simulink library "bcm"  (R2021b)
settings: Solver=VariableStepAuto  StartTime=0.0  StopTime=10.0  RelTol=1e-3
undefined symbols (not defined in the file or in its folder): KBCM_BSDFlashOFFT_cnt, KBCM_BSDFlashONT_cnt, KBCM_BSDRedMode_enum, KBCM_BSDWarnReqLv_enum, KBCM_FireBuzzerEN_flg, KBCM_FLTurnLPLv_A, KBCM_FRTurnLPLv_A, KBCM_LampOFFV_V, KBCM_LampONV_V, KBCM_LightDelayOFFT_Cnt, KBCM_LightDelayONT_Cnt, KBCM_RLTurnLPLv_A, KBCM_RRTurnLPLv_A
libraries: simulink x103, hdlsllib x1
(part 1 of 3)
settings Model: Creator=user  LastModifiedBy=FVT22063
settings SolverCC: AlgebraicLoopSolver=TrustRegion
settings DebuggingCC: SFMachineParentedDataDiag=warning

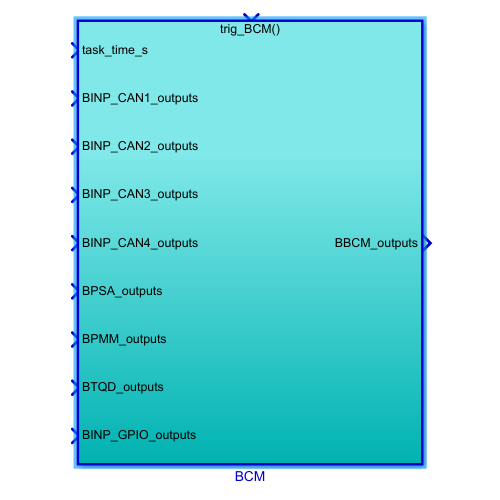
[thumbnail: Simulink's stored preview of the top-level diagram]
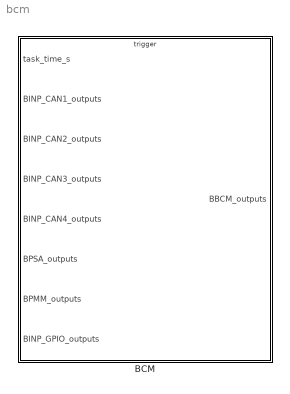
== system bcm ==
  BCM : Subsystem  TreatAsAtomicUnit=on
      settings: RTWSystemCode=Nonreusable function  RTWFcnNameOpts=Use subsystem name  RTWFileNameOpts=Use subsystem name

== system bcm/BCM ==
  note: WarnLv/Mode will be updated on CMM next ver
  note: (Reserved)
      | Actual hazardSW is combinded by L/RTurnSW
  task_time_s : Inport
  BINP_CAN1_outputs : Inport  Port=2  OutDataTypeStr=Bus: BINP_CAN1_outputs
  BINP_CAN2_outputs : Inport  Port=3  OutDataTypeStr=Bus: BINP_CAN2_outputs
  BINP_CAN3_outputs : Inport  Port=4  OutDataTypeStr=Bus: BINP_CAN3_outputs
  BINP_CAN4_outputs : Inport  Port=5  OutDataTypeStr=Bus: BINP_CAN4_outputs
  BPSA_outputs : Inport  Port=6  OutDataTypeStr=Bus: BPSA_outputs
  BPMM_outputs : Inport  Port=7  OutDataTypeStr=Bus: BPMM_outputs
  BINP_GPIO_outputs : Inport  Port=8  OutDataTypeStr=Bus: BINP_GPIO_outputs
  trig_BCM : TriggerPort  TriggerType=function-call  VariantControl=(inherit)
  BBCM_outputs33 : BusCreator  Inputs=56  OutDataTypeStr=Bus: BBCM_outputs  NonVirtualBus=on
  Bus Selector1 : BusSelector  OutputSignals=VINP_EmergencyExitSW_flg,VINP_OSDoorSwOpen_flg,VINP_OSDoorSwClose_flg,VINP_RightTurnSW_flg,VINP_LeftTurnSW_flg
  Bus Selector15 : BusSelector  OutputSignals=VPSA_Keystatus_enum
  Bus Selector16 : BusSelector  OutputSignals=VINP_ZFRBCMHeadLpSWSta_flg,VINP_ZFRBCMHBeamSWSta_flg,VINP_ZFRBCMAutoLightSWSta_flg,VINP_ZFRBCMLightSensorVSta_V,VINP_ZFRBCMPLampSta_flg,VINP_ZFRBCMLFTurnLpCSta_A,VINP_ZFRBCMRFTurnLpCSta_A,VINP_ZRRBCMLRTurnLpCSta_A,VINP_ZRRBCMRRTurnLpCSta_A,VINP_ZRRBCMSTOPSWSta_flg,VINP_ZRRBCMSTOPSW2Sta_flg,VINP_ZRRBCMCallingSWSta_flg,VINP_ZFRBCMWiperASSta_flg,VINP_ZFRBCMWiperHSWSta_flg,VINP_ZFRBCMWiperLSWSta_flg,VINP_ZFRBCMWasherSWSta_flg,VINP_ZFRBCMRFogLpSWSta_flg
  Bus Selector17 : BusSelector  OutputSignals=VPMM_HVILFail_flg
  Bus Selector18 : BusSelector  OutputSignals=VINP_FASpeed_kph,VINP_EBSBrakeSw_enum
  Bus Selector19 : BusSelector  OutputSignals=VINP_B2VFaultCode_enum
  Cast To Boolean : DataTypeConversion  OutDataTypeStr=boolean
  Ground : Ground
  Model Info : simulink/Model-Wide Utilities/Model Info  Frame=on  DisplayStringWithTags=$Id: pmm.mdl 130 2021-02-08 12:40:01Z Shawn $  HorizontalTextAlignment=Center  LeftAlignmentValue=0.5
  Subsystem : Subsystem
  Terminator1 : Terminator
  BBCM_outputs : Outport  OutDataTypeStr=Bus: BBCM_outputs  VectorParamsAs1DForOutWhenUnconnected=off
  wires:
  BPSA_outputs/1 -> Bus Selector15/1
  Bus Selector15/1 -> Subsystem/1(VPMM_VCUKeyStatus_enum)  "<VPSA_Keystatus_enum>"
  BINP_CAN4_outputs/1 -> Bus Selector16/1
  Bus Selector16/1 -> Subsystem/3(VINP_ZFRBCMHeadLpSWSta_flg)  "<VINP_ZFRBCMHeadLpSWSta_flg>"
  Bus Selector16/2 -> Subsystem/4(VINP_ZFRBCMHBeamSWSta_flg)  "<VINP_ZFRBCMHBeamSWSta_flg>"
  Bus Selector16/3 -> Subsystem/5(VINP_ZFRBCMAutoLightSWSta_flg)  "<VINP_ZFRBCMAutoLightSWSta_flg>"
  Bus Selector16/4 -> Subsystem/6(VINP_ZFRBCMLightSensorVSta_V)  "<VINP_ZFRBCMLightSensorVSta_V>"
  Bus Selector16/5 -> Subsystem/7(VINP_ZFRBCMPosLpSWSta_flg)  "<VINP_ZFRBCMPLampSta_flg>"
  Bus Selector16/6 -> Subsystem/8(VINP_ZFRBCMLFTurnLpCSta_A)  "<VINP_ZFRBCMLFTurnLpCSta_A>"
  Bus Selector16/7 -> Subsystem/9(VINP_ZFRBCMRFTurnLpCSta_A)  "<VINP_ZFRBCMRFTurnLpCSta_A>"
  Bus Selector16/8 -> Subsystem/10(VINP_ZRRBCMLRTurnLpCSta_A)  "<VINP_ZRRBCMLRTurnLpCSta_A>"
  Bus Selector16/9 -> Subsystem/11(VINP_ZRRBCMRRTurnLpCSta_A)  "<VINP_ZRRBCMRRTurnLpCSta_A>"
  Ground/1 -> Cast To Boolean/1
  Cast To Boolean/1 -> Subsystem/59(VINP_HazardSW_flg)
  BPMM_outputs/1 -> Bus Selector17/1
  Bus Selector17/1 -> Subsystem/2(VINP_VCUHVILSta_flg)  "<VPMM_HVILFail_flg>"
  Bus Selector16/10 -> Subsystem/12(VINP_ZRRBCMSTOPSWSta_flg)  "<VINP_ZRRBCMSTOPSWSta_flg>"
  Bus Selector16/11 -> Subsystem/13(VINP_ZRRBCMSTOPSW2Sta_flg)  "<VINP_ZRRBCMSTOPSW2Sta_flg>"
  Bus Selector16/12 -> Subsystem/14(VINP_ZRRBCMCallingSWSta_flg)  "<VINP_ZRRBCMCallingSWSta_flg>"
  Bus Selector16/13 -> Subsystem/15(VINP_ZFRBCMWiperASSta_flg)  "<VINP_ZFRBCMWiperASSta_flg>"
  Bus Selector16/14 -> Subsystem/16(VINP_ZFRBCMWiperHSWSta_flg)  "<VINP_ZFRBCMWiperHSWSta_flg>"
  Bus Selector16/15 -> Subsystem/17(VINP_ZFRBCMWiperLSWSta_flg)  "<VINP_ZFRBCMWiperLSWSta_flg>"
  Bus Selector16/16 -> Subsystem/18(VINP_ZFRBCMWasherSWSta_flg)  "<VINP_ZFRBCMWasherSWSta_flg>"
  Bus Selector16/17 -> Subsystem/19(VINP_ZFRBCMRFogLpSWSta_flg)  "<VINP_ZFRBCMRFogLpSWSta_flg>"
  BINP_CAN1_outputs/1 -> Bus Selector18/1
  Bus Selector18/1 -> Subsystem/32(VDIP_VCUVehSpd_kph)  "<VINP_FASpeed_kph>"
  BINP_CAN3_outputs/1 -> Bus Selector19/1
  Bus Selector19/1 -> Subsystem/35(VINP_B2VFaultCode_enum)  "<VINP_B2VFaultCode_enum>"
  Bus Selector18/2 -> Subsystem/33(VINP_EBSBrakeSw_flg)  "<VINP_EBSBrakeSw_enum>"
  BINP_CAN2_outputs/1 -> Terminator1/1
  BINP_GPIO_outputs/1 -> Bus Selector1/1
  BBCM_outputs33/1 -> BBCM_outputs/1
  Subsystem/1(VBCM_FDCBCMLBeamCmd_flg) -> BBCM_outputs33/1  "VBCM_FDCBCMLBeamCmd_flg"
  Subsystem/2(VBCM_FDCBCMPLampCmd_flg) -> BBCM_outputs33/2  "VBCM_FDCBCMPLampCmd_flg"
  Subsystem/3(VBCM_FDCBCMHBeamCmd_flg) -> BBCM_outputs33/3  "VBCM_FDCBCMHBeamCmd_flg"
  Subsystem/4(VBCM_FDCBCMSMKLCmd_flg) -> BBCM_outputs33/4  "VBCM_FDCBCMSMKLCmd_flg"
  Subsystem/5(VBCM_FDCBCMSMKRCmd_flg) -> BBCM_outputs33/5  "VBCM_FDCBCMSMKRCmd_flg"
  Subsystem/6(VBCM_FDCBCMDVRSignalLCmd_flg) -> BBCM_outputs33/6  "VBCM_FDCBCMDVRSignalLCmd_flg"
  Subsystem/7(VBCM_FDCBCMDVRSignalRCmd_flg) -> BBCM_outputs33/7  "VBCM_FDCBCMDVRSignalRCmd_flg"
  Subsystem/8(VBCM_FDCBCMBSDBuzzerCmd_flg) -> BBCM_outputs33/8  "VBCM_FDCBCMBSDBuzzerCmd_flg"
  Subsystem/9(VBCM_FDCBCMSLTLpCmd_flg) -> BBCM_outputs33/9  "VBCM_FDCBCMSLTLpCmd_flg"
  Subsystem/10(VBCM_FDCBCMSRTLpCmd_flg) -> BBCM_outputs33/10  "VBCM_FDCBCMSRTLpCmd_flg"
  Subsystem/11(VBCM_FDCBCMLTurnLpCmd_flg) -> BBCM_outputs33/11  "VBCM_FDCBCMLTurnLpCmd_flg"
  Subsystem/12(VBCM_FDCBCMRTurnLpCmd_flg) -> BBCM_outputs33/12  "VBCM_FDCBCMRTurnLpCmd_flg"
  Subsystem/13(VBCM_FDCBCMStopINDCmd_flg) -> BBCM_outputs33/13  "VBCM_FDCBCMStopINDCmd_flg"
  Subsystem/14(VBCM_FDCBCMSTOPBALLCmd_flg) -> BBCM_outputs33/14  "VBCM_FDCBCMSTOPBALLCmd_flg"
  Subsystem/15(VBCM_FDCBCMInnerCallBellCmd_flg) -> BBCM_outputs33/15  "VBCM_FDCBCMInnerCallBellCmd_flg"
  Subsystem/16(VBCM_FDCBCMCallBellCmd_flg) -> BBCM_outputs33/16  "VBCM_FDCBCMCallBellCmd_flg"
  Subsystem/17(VBCM_FDCBCMWiperHCmd_flg) -> BBCM_outputs33/17  "VBCM_FDCBCMWiperHCmd_flg"
  Subsystem/18(VBCM_FDCBCMWasherCmd_flg) -> BBCM_outputs33/18  "VBCM_FDCBCMWasherCmd_flg"
  Subsystem/19(VBCM_FDCBCMWiperLCmd_flg) -> BBCM_outputs33/19  "VBCM_FDCBCMWiperLCmd_flg"
  Subsystem/20(VBCM_FDCBCMLDRLCmd_flg) -> BBCM_outputs33/20  "VBCM_FDCBCMLDRLCmd_flg"
  Subsystem/21(VBCM_FDCBCMRDRLCmd_flg) -> BBCM_outputs33/21  "VBCM_FDCBCMRDRLCmd_flg"
  Subsystem/22(VBCM_FDCBCMRFLampCmd_flg) -> BBCM_outputs33/22  "VBCM_FDCBCMRFLampCmd_flg"
  Subsystem/23(VBCM_FDCBCMTurnLpPatternSta_enum) -> BBCM_outputs33/23  "VBCM_TurnLpPatternSta_enum"
  Subsystem/24(VBCM_FDCBCMFDoorSta_flg) -> BBCM_outputs33/24  "VBCM_FDCBCMFDoorSta_flg"
  Subsystem/25(VBCM_FDCBCMMDoorSta_flg) -> BBCM_outputs33/25  "VBCM_FDCBCMMDoorSta_flg"
  Subsystem/26(VBCM_FDCBCMRDoorSta_flg) -> BBCM_outputs33/26  "VBCM_FDCBCMRDoorSta_flg"
  Subsystem/27(VBCM_FDCBCMRoomLpAmbCmd_flg) -> BBCM_outputs33/27  "VBCM_FDCBCMRoomLpAmbCmd_flg"
  Subsystem/28(VBCM_FDCBCMLBSDRCmd_flg) -> BBCM_outputs33/28  "VBCM_FDCBCMLBSDRCmd_flg"
  Subsystem/29(VBCM_FDCBCMLBSDYCmd_flg) -> BBCM_outputs33/29  "VBCM_FDCBCMLBSDYCmd_flg"
  Subsystem/30(VBCM_FDCBCMRBSDRCmd_flg) -> BBCM_outputs33/30  "VBCM_FDCBCMRBSDRCmd_flg"
  Subsystem/31(VBCM_FDCBCMRBSDYCmd_flg) -> BBCM_outputs33/31  "VBCM_FDCBCMRBSDYCmd_flg"
  Subsystem/32(VBCM_FDCBCMEmExitSWSta_flg) -> BBCM_outputs33/32  "VBCM_FDCBCMEmExitSWSta_flg"
  Subsystem/33(VBCM_FDCBCMInnerBuzzerModeSta_enum) -> BBCM_outputs33/33  "VBCM_InnerBuzzerModeSta_enum"
  Subsystem/34(VBCM_FDCBCMInnerBuzzerCmd_flg) -> BBCM_outputs33/34  "VBCM_FDCBCMInnerBuzzerCmd_flg"
  Subsystem/35(VBCM_FDCBCMRoomLpAmbSetSta_flg) -> BBCM_outputs33/35  "VBCM_FDCBCMRoomLpAmbSetSta_flg"
  Subsystem/36(VBCM_FDCBCMRoomLpSetSta_flg) -> BBCM_outputs33/36  "VBCM_FDCBCMRoomLpSetSta_flg"
  Subsystem/37(VBCM_FDCBCMFRoomLpSetSta_pct) -> BBCM_outputs33/37  "VBCM_FDCBCMFRoomLpSetSta_pct"
  Subsystem/38(VBCM_FDCBCMFRoomLpCmd_pct) -> BBCM_outputs33/38  "VBCM_FDCBCMFRoomLpCmd_pct"
  Subsystem/39(VBCM_FDCBCMMRoomLpSetSta_pct) -> BBCM_outputs33/39  "VBCM_FDCBCMMRoomLpSetSta_pct"
  Subsystem/40(VBCM_FDCBCMMRoomLpCmd_pct) -> BBCM_outputs33/40  "VBCM_FDCBCMMRoomLpCmd_pct"
  Subsystem/41(VBCM_FDCBCMRRoomLpSetSta_pct) -> BBCM_outputs33/41  "VBCM_FDCBCMRRoomLpSetSta_pct"
  Subsystem/42(VBCM_FDCBCMRRoomLpCmd_pct) -> BBCM_outputs33/42  "VBCM_FDCBCMRRoomLpCmd_pct"
  Subsystem/43(VBCM_FDCBCMHelpINDCmd_flg) -> BBCM_outputs33/43  "VBCM_FDCBCMHelpINDCmd_flg"
  Subsystem/44(VBCM_FDCBCMOSDrOpenSWSta_enum) -> BBCM_outputs33/44  "VBCM_FDCBCMOSDrOpenSWSta_enum"
  Subsystem/45(VBCM_FDCBCMEmSVCmd_flg) -> BBCM_outputs33/45  "VBCM_FDCBCMEmSVCmd_flg"
  Subsystem/46(VBCM_FDCBCMFDOpenSVCmd_flg) -> BBCM_outputs33/46  "VBCM_FDCBCMFDOpenSVCmd_flg"
  Subsystem/47(VBCM_FDCBCMFDCloseSVCmd_flg) -> BBCM_outputs33/47  "VBCM_FDCBCMFDCloseSVCmd_flg"
  Subsystem/48(VBCM_FDCBCMMDOpenSVCmd_flg) -> BBCM_outputs33/48  "VBCM_FDCBCMMDOpenSVCmd_flg"
  Subsystem/49(VBCM_FDCBCMMDCloseSVCmd_flg) -> BBCM_outputs33/49  "VBCM_FDCBCMMDCloseSVCmd_flg"
  Subsystem/50(VBCM_FDCBCMLTurnSWSta_flg) -> BBCM_outputs33/50  "VBCM_FDCBCMLTurnSWSta_flg"
  Subsystem/51(VBCM_FDCBCMRTurnSWSta_flg) -> BBCM_outputs33/51  "VBCM_FDCBCMRTurnSWSta_flg"
  Subsystem/52(VBCM_FDCBCMRGearSta_flg) -> BBCM_outputs33/52  "VBCM_FDCBCMRGearSta_flg"
  Subsystem/53(VBCM_FDCBCMBrakeCmd_flg) -> BBCM_outputs33/53  "VBCM_FDCBCMBrakeCmd_flg"
  Subsystem/54(VBCM_FDCBCMTurnBuzzerENSta_flg) -> BBCM_outputs33/54  "VBCM_FDCBCMTurnBuzzerENSta_flg"
  Subsystem/55(VBCM_WakeUp_flg) -> BBCM_outputs33/55  "VBCM_WakeUp_flg"
  Subsystem/56(VBCM_KeepWakeUp_flg) -> BBCM_outputs33/56  "VBCM_KeepWakeUp_flg"
  Bus Selector1/5 -> Subsystem/58(VINP_LTurnSW_flg)  "<VINP_LeftTurnSW_flg>"
  Bus Selector1/4 -> Subsystem/57(VINP_RTurnSW_flg)  "<VINP_RightTurnSW_flg>"
  Bus Selector1/3 -> Subsystem/56(VINP_OSDoorCloseSW_flg)  "<VINP_OSDoorSwClose_flg>"
  Bus Selector1/2 -> Subsystem/55(VINP_OSDoorOpenSW_flg)  "<VINP_OSDoorSwOpen_flg>"
  Bus Selector1/1 -> Subsystem/54(VINP_EmExitSW_flg)  "<VINP_EmergencyExitSW_flg>"

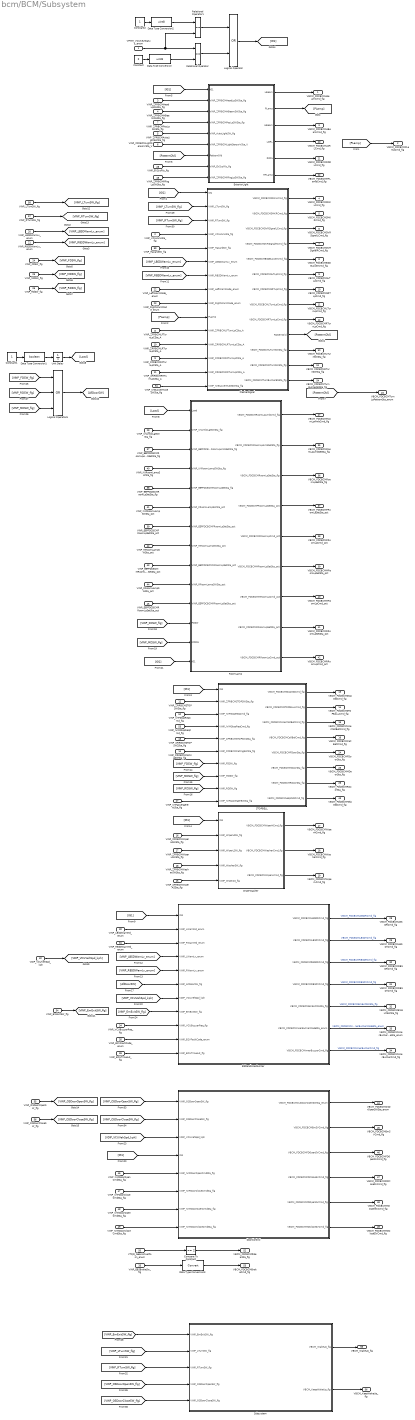
== system bcm/BCM/Subsystem ==
  VPMM_VCUKeyStatus_enum : Inport
  VINP_VCUHVILSta_flg : Inport  Port=2
  VINP_ZFRBCMHeadLpSWSta_flg : Inport  Port=3
  VINP_ZFRBCMHBeamSWSta_flg : Inport  Port=4
  VINP_ZFRBCMAutoLightSWSta_flg : Inport  Port=5
  VINP_ZFRBCMLightSensorVSta_V : Inport  Port=6
  VINP_ZFRBCMPosLpSWSta_flg : Inport  Port=7
  VINP_ZFRBCMLFTurnLpCSta_A : Inport  Port=8
  VINP_ZFRBCMRFTurnLpCSta_A : Inport  Port=9
  VINP_ZRRBCMLRTurnLpCSta_A : Inport  Port=10
  VINP_ZRRBCMRRTurnLpCSta_A : Inport  Port=11
  VINP_ZRRBCMSTOPSWSta_flg : Inport  Port=12
  VINP_ZRRBCMSTOPSW2Sta_flg : Inport  Port=13
  VINP_ZRRBCMCallingSWSta_flg : Inport  Port=14
  VINP_ZFRBCMWiperASSta_flg : Inport  Port=15
  VINP_ZFRBCMWiperHSWSta_flg : Inport  Port=16
  VINP_ZFRBCMWiperLSWSta_flg : Inport  Port=17
  VINP_ZFRBCMWasherSWSta_flg : Inport  Port=18
  VINP_ZFRBCMRFogLpSWSta_flg : Inport  Port=19
  VINP_LBSDWarnLv_enum : Inport  Port=20
  VINP_RBSDWarnLv_enum : Inport  Port=21
  VINP_LeftWarnMode_enum : Inport  Port=22
  VINP_RightWarnMode_enum : Inport  Port=23
  VINP_FDSW_flg : Inport  Port=24
  VINP_MDSW_flg : Inport  Port=25
  VINP_RDSW_flg : Inport  Port=26
  VINP_IVIPassengerExtSta_flg : Inport  Port=27
  VINP_EVSysRls_flg : Inport  Port=28
  VINP_IVIAmbiLgtSWSta_flg : Inport  Port=29
  VINP_LBSDWarnMd_enum : Inport  Port=30
  VINP_RBSDWarnMd_enum : Inport  Port=31
  VDIP_VCUVehSpd_kph : Inport  Port=32
  VINP_EBSBrakeSw_flg : Inport  Port=33
  VINP_VCUBuzzerReq_flg : Inport  Port=34
  VINP_B2VFaultCode_enum : Inport  Port=35
  VINP_BCUTimeout_flg : Inport  Port=36
  VINP_EEPFDCBCMRoomLpAmbSetSta_flg : Inport  Port=37
  VINP_EEPFDCBCMRoomLpSetSta_flg : Inport  Port=38
  VINP_EEPFDCBCMFRoomLpSetSta_pct : Inport  Port=39
  VINP_IVIRoomLampSWSta_flg : Inport  Port=40
  VINP_IVIFRoomLampSWSta_pct : Inport  Port=41
  VINP_MRoomLampSWSta_pct : Inport  Port=42
  VINP_EEPFDCBCMMRoomLpSetSta_pct : Inport  Port=43
  VINP_RRoomLampSWSta_pct : Inport  Port=44
  VINP_EEPFDCBCMRRoomLpSetSta_pct : Inport  Port=45
  VINP_IVIFDoorOpenCmdSta_flg : Inport  Port=46
  VINP_IVIFDoorCloseCmdSta_flg : Inport  Port=47
  VINP_IVIMDoorOpenCmdSta_flg : Inport  Port=48
  VINP_IVIMDoorCloseCmdSta_flg : Inport  Port=49
  VTQD_GearActualPosn_enum : Inport  Port=50
  VINP_IVIBuzzerMuteSWSta_flg : Inport  Port=51
  VINP_IVIFStopReqCmd_flg : Inport  Port=52
  VINP_IVIMStopReqCmd_flg : Inport  Port=53
  VINP_EmExitSW_flg : Inport  Port=54
  VINP_OSDoorOpenSW_flg : Inport  Port=55
  VINP_OSDoorCloseSW_flg : Inport  Port=56
  VINP_RTurnSW_flg : Inport  Port=57
  VINP_LTurnSW_flg : Inport  Port=58
  VINP_HazardSW_flg : Inport  Port=59
  BSDandInnerBuzzer : Subsystem
  Compare To Constant : simulink/Logic and Bit Operations/Compare To Constant  relop===  const=2  OutDataTypeStr=boolean
  Constant : Constant  Value=2
  Constant1 : Constant
  Constant2 : Constant
  Data Type Conversion : DataTypeConversion  OutDataTypeStr=uint8
  Data Type Conversion1 : DataTypeConversion  OutDataTypeStr=boolean
  Data Type Conversion2 : DataTypeConversion  OutDataTypeStr=uint8
  Data Type Conversion3 : DataTypeConversion
  DoorControl : Subsystem
  ExteriorLight : Subsystem
  FlasherSignal : Subsystem
  Logical Operator : Logic  Operator=OR  AllPortsSameDT=off  OutDataTypeStr=boolean
  Logical Operator6 : Logic  Operator=OR  Inputs=3  AllPortsSameDT=off  OutDataTypeStr=boolean
  Relational Operator : RelationalOperator  Operator===  OutDataTypeStr=boolean  RndMeth=Simplest
  Relational Operator1 : RelationalOperator  Operator===  OutDataTypeStr=boolean  RndMeth=Simplest
  RoomLamp : Subsystem
  STOPBELL : Subsystem
  Subsystem : Subsystem
  Unit Delay : UnitDelay  SampleTime=-1  HasFrameUpgradeWarning=on
  WiperWasher : Subsystem
  VBCM_FDCBCMLBeamCmd_flg : Outport
  VBCM_FDCBCMPLampCmd_flg : Outport  Port=2
  VBCM_FDCBCMHBeamCmd_flg : Outport  Port=3
  VBCM_FDCBCMSMKLCmd_flg : Outport  Port=4
  VBCM_FDCBCMSMKRCmd_flg : Outport  Port=5
  VBCM_FDCBCMDVRSignalLCmd_flg : Outport  Port=6
  VBCM_FDCBCMDVRSignalRCmd_flg : Outport  Port=7
  VBCM_FDCBCMBSDBuzzerCmd_flg : Outport  Port=8
  VBCM_FDCBCMSLTLpCmd_flg : Outport  Port=9
  VBCM_FDCBCMSRTLpCmd_flg : Outport  Port=10
  VBCM_FDCBCMLTurnLpCmd_flg : Outport  Port=11
  VBCM_FDCBCMRTurnLpCmd_flg : Outport  Port=12
  VBCM_FDCBCMStopINDCmd_flg : Outport  Port=13
  VBCM_FDCBCMSTOPBALLCmd_flg : Outport  Port=14
  VBCM_FDCBCMInnerCallBellCmd_flg : Outport  Port=15
  VBCM_FDCBCMCallBellCmd_flg : Outport  Port=16
  VBCM_FDCBCMWiperHCmd_flg : Outport  Port=17
  VBCM_FDCBCMWasherCmd_flg : Outport  Port=18
  VBCM_FDCBCMWiperLCmd_flg : Outport  Port=19
  VBCM_FDCBCMLDRLCmd_flg : Outport  Port=20
  VBCM_FDCBCMRDRLCmd_flg : Outport  Port=21
  VBCM_FDCBCMRFLampCmd_flg : Outport  Port=22
  VBCM_FDCBCMTurnLpPatternSta_enum : Outport  Port=23
  VBCM_FDCBCMFDoorSta_flg : Outport  Port=24
  VBCM_FDCBCMMDoorSta_flg : Outport  Port=25
  VBCM_FDCBCMRDoorSta_flg : Outport  Port=26
  VBCM_FDCBCMRoomLpAmbCmd_flg : Outport  Port=27
  VBCM_FDCBCMLBSDRCmd_flg : Outport  Port=28
  VBCM_FDCBCMLBSDYCmd_flg : Outport  Port=29
  VBCM_FDCBCMRBSDRCmd_flg : Outport  Port=30
  VBCM_FDCBCMRBSDYCmd_flg : Outport  Port=31
  VBCM_FDCBCMEmExitSWSta_flg : Outport  Port=32
  VBCM_FDCBCMInnerBuzzerModeSta_enum : Outport  Port=33
  VBCM_FDCBCMInnerBuzzerCmd_flg : Outport  Port=34
  VBCM_FDCBCMRoomLpAmbSetSta_flg : Outport  Port=35
  VBCM_FDCBCMRoomLpSetSta_flg : Outport  Port=36
  VBCM_FDCBCMFRoomLpSetSta_pct : Outport  Port=37
  VBCM_FDCBCMFRoomLpCmd_pct : Outport  Port=38
  VBCM_FDCBCMMRoomLpSetSta_pct : Outport  Port=39
  VBCM_FDCBCMMRoomLpCmd_pct : Outport  Port=40
  VBCM_FDCBCMRRoomLpSetSta_pct : Outport  Port=41
  VBCM_FDCBCMRRoomLpCmd_pct : Outport  Port=42
  VBCM_FDCBCMHelpINDCmd_flg : Outport  Port=43
  VBCM_FDCBCMOSDrOpenSWSta_enum : Outport  Port=44
  VBCM_FDCBCMEmSVCmd_flg : Outport  Port=45
  VBCM_FDCBCMFDOpenSVCmd_flg : Outport  Port=46
  VBCM_FDCBCMFDCloseSVCmd_flg : Outport  Port=47
  VBCM_FDCBCMMDOpenSVCmd_flg : Outport  Port=48
  VBCM_FDCBCMMDCloseSVCmd_flg : Outport  Port=49
  VBCM_FDCBCMLTurnSWSta_flg : Outport  Port=50
  VBCM_FDCBCMRTurnSWSta_flg : Outport  Port=51
  VBCM_FDCBCMRGearSta_flg : Outport  Port=52
  VBCM_FDCBCMBrakeCmd_flg : Outport  Port=53
  VBCM_FDCBCMTurnBuzzerENSta_flg : Outport  Port=54
  VBCM_WakeUp_flg : Outport  Port=55
  VBCM_KeepWakeUp_flg : Outport  Port=56
  wires:
  VINP_RBSDWarnMd_enum/1 -> BSDandInnerBuzzer/3(VINP_RWarnMd_enum)
  Compare To Constant/1 -> VBCM_FDCBCMRGearSta_flg/1
  ExteriorLight/5(RDRL) -> VBCM_FDCBCMRDRLCmd_flg/1
  RoomLamp/8(VBCM_FDCBCMRRoomLpSetSta_pct) -> VBCM_FDCBCMRRoomLpSetSta_pct/1
  VINP_IVIPassengerExtSta_flg/1 -> STOPBELL/10(VINP_IVIPassengerExtSta_flg)
  BSDandInnerBuzzer/7(VBCM_FDCBCMInnerBuzzerCmd_flg) -> VBCM_FDCBCMInnerBuzzerCmd_flg/1  "VBCM_FDCBCMInnerBuzzerCmd_flg"
  FlasherSignal/9(VBCM_FDCBCMRTurnLpCmd_flg) -> VBCM_FDCBCMRTurnLpCmd_flg/1
  Data Type Conversion/1 -> Relational Operator/2
  Subsystem/1(VBCM_WakeUp_flg) -> VBCM_WakeUp_flg/1
  VINP_RTurnSW_flg/1 -> [VINP_RTurnSW_flg]
  VINP_VCUHVILSta_flg/1 -> FlasherSignal/4(VINP_VCUHVILSta_flg)
  FlasherSignal/8(VBCM_FDCBCMLTurnLpCmd_flg) -> VBCM_FDCBCMLTurnLpCmd_flg/1
  VINP_EBSBrakeSw_flg/1 -> Data Type Conversion3/1
  ExteriorLight/4(LDRL) -> VBCM_FDCBCMLDRLCmd_flg/1
  STOPBELL/2(VBCM_FDCBCMSTOPBALLCmd_flg) -> VBCM_FDCBCMSTOPBALLCmd_flg/1
  VINP_RightWarnMode_enum/1 -> FlasherSignal/9(VINP_RightWarnMode_enum)
  [PatternOld] -> VBCM_FDCBCMTurnLpPatternSta_enum/1
  BSDandInnerBuzzer/3(VBCM_FDCBCMRBSDRCmd_flg) -> VBCM_FDCBCMRBSDRCmd_flg/1  "VBCM_FDCBCMRBSDRCmd_flg"
  FlasherSignal/7(VBCM_FDCBCMSRTLpCmd_flg) -> VBCM_FDCBCMSRTLpCmd_flg/1
  [VINP_OSDoorOpenSW_flg] -> Subsystem/4(VINP_OSDoorOpenSW_flg)
  VINP_ZFRBCMAutoLightSWSta_flg/1 -> ExteriorLight/5(VINP_AutoLightSW_flg)
  Subsystem/2(VBCM_KeepWakeUp_flg) -> VBCM_KeepWakeUp_flg/1
  RoomLamp/9(VBCM_FDCBCMRRoomLpCmd_pct) -> VBCM_FDCBCMRRoomLpCmd_pct/1
  [VINP_RTurnSW_flg] -> FlasherSignal/3(VINP_RTurnSW_flg)
  [VINP_LBSDWarnLv_enum] -> BSDandInnerBuzzer/4(VINP_LWarnLv_enum)
  Unit Delay/1 -> [Load]
  VDIP_VCUVehSpd_kph/1 -> [VDIP_VCUVehSpd_kph]
  DoorControl/3(VBCM_FDCBCMFDOpenSVCmd_flg) -> VBCM_FDCBCMFDOpenSVCmd_flg/1
  [VINP_EmExitSW_flg] -> BSDandInnerBuzzer/8(VINP_EmExitSW_flg)
  FlasherSignal/5(VBCM_FDCBCMBSDBuzzerCmd_flg) -> VBCM_FDCBCMBSDBuzzerCmd_flg/1
  VINP_LBSDWarnMd_enum/1 -> BSDandInnerBuzzer/2(VINP_LWarnMd_enum)
  [VINP_LTurnSW_flg] -> Subsystem/2(VINP_LTurnSW_flg)
  VINP_OSDoorOpenSW_flg/1 -> [VINP_OSDoorOpenSW_flg]
  Logical Operator6/1 -> [AllDoorSW]
  VINP_ZFRBCMHeadLpSWSta_flg/1 -> ExteriorLight/2(VINP_ZFRBCMHeadLpSWSta_flg)
  [IG1] -> FlasherSignal/1(IG1)
  FlasherSignal/10(PatternOld) -> [PatternOld]
  VINP_RBSDWarnLv_enum/1 -> [VINP_RBSDWarnLv_enum]
  RoomLamp/4(VBCM_FDCBCMFRoomLpSetSta_pct) -> VBCM_FDCBCMFRoomLpSetSta_pct/1
  [VINP_RDSW_flg] -> Logical Operator6/2
  VINP_ZFRBCMPosLpSWSta_flg/1 -> ExteriorLight/4(VINP_ZFRBCMPosLpSWSta_flg)
  VINP_IVIMDoorCloseCmdSta_flg/1 -> DoorControl/8(VINP_IVIMDoorCloseCmdSta_flg)
  VINP_ZFRBCMWasherSWSta_flg/1 -> WiperWasher/4(VINP_WasherSW_flg)
  VINP_ZFRBCMLightSensorVSta_V/1 -> ExteriorLight/6(VINP_ZFRBCMLightSensorVSta_V)
  VINP_VCUBuzzerReq_flg/1 -> BSDandInnerBuzzer/9(VINP_VCUBuzzerReq_flg)
  VINP_ZFRBCMRFogLpSWSta_flg/1 -> ExteriorLight/9(VINP_ZFRBCMRFogLpSWSta_flg)
  STOPBELL/4(VBCM_FDCBCMCallBelCmd_flg) -> VBCM_FDCBCMCallBellCmd_flg/1
  VINP_IVIMStopReqCmd_flg/1 -> STOPBELL/4(VINP_IVIMStopReqCmd_flg)
  VINP_MDSW_flg/1 -> [VINP_MDSW_flg]
  VINP_IVIFDoorOpenCmdSta_flg/1 -> DoorControl/5(VINP_IVIFDoorOpenCmdSta_flg)
  VINP_EEPFDCBCMRoomLpSetSta_flg/1 -> RoomLamp/5(VINP_EEPFDCBCMRoomLpSetSta_flg)
  STOPBELL/6(VBCM_FDCBCMMDoorSta_flg) -> VBCM_FDCBCMMDoorSta_flg/1
  VINP_ZFRBCMWiperLSWSta_flg/1 -> WiperWasher/3(VINP_WiperLSW_flg)
  DoorControl/2(VBCM_FDCBCMEmSVCmd_flg) -> VBCM_FDCBCMEmSVCmd_flg/1
  [VINP_FDSW_flg] -> STOPBELL/7(VINP_FDSW_flg)
  STOPBELL/8(VBCM_FDCBCMHelpINDCmd_flg) -> VBCM_FDCBCMHelpINDCmd_flg/1
  VINP_OSDoorCloseSW_flg/1 -> [VINP_OSDoorCloseSW_flg]
  [VINP_RTurnSW_flg] -> Subsystem/3(VINP_RTurnSW_flg)
  VINP_LTurnSW_flg/1 -> [VINP_LTurnSW_flg]
  BSDandInnerBuzzer/5(VBCM_FDCBCMEmExitSWSta_flg) -> VBCM_FDCBCMEmExitSWSta_flg/1  "VBCM_FDCBCMEmExitSWSta_flg"
  ExteriorLight/3(HBeam) -> VBCM_FDCBCMHBeamCmd_flg/1
  [IG1] -> ExteriorLight/1(IG1)
  [Load] -> RoomLamp/1(Load)
  [PLamp] -> FlasherSignal/10(PLamp)
  VINP_EEPFDCBCMFRoomLpSetSta_pct/1 -> RoomLamp/7(VINP_EEPFDCBCMFRoomLpSetSta_pct)
  DoorControl/5(VBCM_FDCBCMMDOpenSVCmd_flg) -> VBCM_FDCBCMMDOpenSVCmd_flg/1
  VINP_HazardSW_flg/1 -> FlasherSignal/5(VINP_HazardSW_flg)
  VINP_EEPFDCBCMMRoomLpSetSta_pct/1 -> RoomLamp/9(VINP_EEPFDCBCMMRoomLpSetSta_pct)
  BSDandInnerBuzzer/6(VBCM_FDCBCMInnerBuzzerModeSta_enum) -> VBCM_FDCBCMInnerBuzzerModeSta_enum/1  "VBCM_FDCBCMInnerBuzzerModeSta_enum"
  [VINP_OSDoorOpenSW_flg] -> DoorControl/1(VINP_OSDoorOpenSW_flg)
  [VINP_EmExitSW_flg] -> Subsystem/1(VINP_EmExitSW_flg)
  VINP_LBSDWarnLv_enum/1 -> [VINP_LBSDWarnLv_enum]
  STOPBELL/1(VBCM_FDCBCMStopINDCmd_flg) -> VBCM_FDCBCMStopINDCmd_flg/1
  FlasherSignal/11(VBCM_FDCBCMLTurnSWSta_flg) -> VBCM_FDCBCMLTurnSWSta_flg/1
  [VDIP_VCUVehSpd_kph] -> DoorControl/3(VDIP_VCUVehSpd_kph)
  FlasherSignal/12(VBCM_FDCBCMRTurnSWSta_flg) -> VBCM_FDCBCMRTurnSWSta_flg/1
  VINP_IVIRoomLampSWSta_flg/1 -> RoomLamp/4(VINP_IVIRoomLampSWSta_flg)
  RoomLamp/5(VBCM_FDCBCMFRoomLpCmd_pct) -> VBCM_FDCBCMFRoomLpCmd_pct/1
  [IG1] -> STOPBELL/1(IG1)
  VINP_ZRRBCMSTOPSWSta_flg/1 -> STOPBELL/2(VINP_ZFRBCMSTOPSWSta_flg)
  VINP_LeftWarnMode_enum/1 -> FlasherSignal/8(VINP_LeftWarnMode_enum)
  BSDandInnerBuzzer/1(VBCM_FDCBCMLBSDRCmd_flg) -> VBCM_FDCBCMLBSDRCmd_flg/1  "VBCM_FDCBCMLBSDRCmd_flg"
  WiperWasher/1(VBCM_FDCBCMWiperHCmd_flg) -> VBCM_FDCBCMWiperHCmd_flg/1
  VINP_IVIFDoorCloseCmdSta_flg/1 -> DoorControl/6(VINP_IVIFDoorCloseCmdSta_flg)
  [VINP_LTurnSW_flg] -> FlasherSignal/2(VINP_LTurnSW_flg)
  [VINP_OSDoorCloseSW_flg] -> Subsystem/5(VINP_OSDoorCloseSW_flg)
  [VINP_OSDoorCloseSW_flg] -> DoorControl/2(VINP_OSDoorCloseSW_flg)
  FlasherSignal/2(VBCM_FDCBCMSMKRCmd_flg) -> VBCM_FDCBCMSMKRCmd_flg/1
  WiperWasher/2(VBCM_FDCBCMWasherCmd_flg) -> VBCM_FDCBCMWasherCmd_flg/1
  FlasherSignal/3(VBCM_FDCBCMDVRSignalLCmd_flg) -> VBCM_FDCBCMDVRSignalLCmd_flg/1
  RoomLamp/3(VBCM_FDCBCMRoomLpSetSta_flg) -> VBCM_FDCBCMRoomLpSetSta_flg/1
  [PLamp] -> VBCM_FDCBCMPLampCmd_flg/1
  [PatternOld] -> ExteriorLight/7(PatternOld)
  VINP_ZFRBCMHBeamSWSta_flg/1 -> ExteriorLight/3(VINP_ZFRBCMHBeamSWSta_flg)
  [VINP_LBSDWarnLv_enum] -> FlasherSignal/6(VINP_LBSDWarnLv_enum)
  [VINP_MDSW_flg] -> RoomLamp/13(MDSW)
  VINP_ZFRBCMWiperHSWSta_flg/1 -> WiperWasher/2(VINP_WiperHSW_flg)
  VPMM_VCUKeyStatus_enum/1 -> Relational Operator1/2, Relational Operator/1
  FlasherSignal/13(VBCM_FDCBCMTurnBuzzerENSta_flg) -> VBCM_FDCBCMTurnBuzzerENSta_flg/1
  [IG1] -> RoomLamp/14(IG1)
  [VINP_MDSW_flg] -> STOPBELL/8(VINP_MDSW_flg)
  VINP_EEPFDCBCMRRoomLpSetSta_pct/1 -> RoomLamp/11(VINP_EEPFDCBCMRRoomLpSetSta_pct)
  [VINP_RBSDWarnLv_enum] -> FlasherSignal/7(VINP_RBSDWarnLv_enum)
  Data Type Conversion1/1 -> Unit Delay/1
  VTQD_GearActualPosn_enum/1 -> Compare To Constant/1
  VINP_IVIBuzzerMuteSWSta_flg/1 -> FlasherSignal/15(VINP_IVIBuzzerMuteSWSta_flg)
  FlasherSignal/6(VBCM_FDCBCMSLTLpCmd_flg) -> VBCM_FDCBCMSLTLpCmd_flg/1
  [VINP_RBSDWarnLv_enum] -> BSDandInnerBuzzer/5(VINP_RWarnLv_enum)
  STOPBELL/5(VBCM_FDCBCMFDoorSta_flg) -> VBCM_FDCBCMFDoorSta_flg/1
  VINP_IVIMDoorOpenCmdSta_flg/1 -> DoorControl/7(VINP_IVIMDoorOpenCmdSta_flg)
  Constant1/1 -> Data Type Conversion1/1
  VINP_MRoomLampSWSta_pct/1 -> RoomLamp/8(VINP_MRoomLampSWSta_pct)
  [IG1] -> WiperWasher/1(IG1)
  ExteriorLight/2(PLamp) -> [PLamp]
  [VINP_RDSW_flg] -> STOPBELL/9(VINP_RDSW_flg)
  FlasherSignal/1(VBCM_FDCBCMSMKLCmd_flg) -> VBCM_FDCBCMSMKLCmd_flg/1
  [IG1] -> DoorControl/4(IG1)
  [AllDoorSW] -> BSDandInnerBuzzer/6(VINP_AllDoorSW_flg)
  [VINP_MDSW_flg] -> Logical Operator6/3
  WiperWasher/3(VBCM_FDCBCMWiperLCmd_flg) -> VBCM_FDCBCMWiperLCmd_flg/1
  FlasherSignal/4(VBCM_FDCBCMDVRSignalRCmd_flg) -> VBCM_FDCBCMDVRSignalRCmd_flg/1
  VINP_FDSW_flg/1 -> [VINP_FDSW_flg]
  STOPBELL/7(VBCM_FDCBCMRDoorSta_flg) -> VBCM_FDCBCMRDoorSta_flg/1
  [VINP_FDSW_flg] -> RoomLamp/12(FDSW)
  VINP_RRoomLampSWSta_pct/1 -> RoomLamp/10(VINP_RRoomLampSWSta_pct)
  VINP_IVIFRoomLampSWSta_pct/1 -> RoomLamp/6(VINP_FRoomLampSWSta_pct)
  VINP_ZFRBCMWiperASSta_flg/1 -> WiperWasher/5(VINP_WiperAS_flg)
  STOPBELL/3(VBCM_FDCBCMInnerCallBellCmd_flg) -> VBCM_FDCBCMInnerCallBellCmd_flg/1
  [VDIP_VCUVehSpd_kph] -> BSDandInnerBuzzer/7(VDIP_VCUVehSpd_kph)
  RoomLamp/6(VBCM_FDCBCMMRoomLpSetSta_pct) -> VBCM_FDCBCMMRoomLpSetSta_pct/1
  VINP_IVIFStopReqCmd_flg/1 -> STOPBELL/3(VINP_IVIFStopReqCmd_flg)
  BSDandInnerBuzzer/4(VBCM_FDCBCMRBSDYCmd_flg) -> VBCM_FDCBCMRBSDYCmd_flg/1  "VBCM_FDCBCMRBSDYCmd_flg"
  BSDandInnerBuzzer/2(VBCM_FDCBCMLBSDYCmd_flg) -> VBCM_FDCBCMLBSDYCmd_flg/1  "VBCM_FDCBCMLBSDYCmd_flg"
  VINP_EVSysRls_flg/1 -> ExteriorLight/8(VINP_EVSysRls_flg)
  VINP_IVIAmbiLgtSWSta_flg/1 -> RoomLamp/2(VINP_IVIAmbiLgtSWSta_flg)
  VINP_ZRRBCMSTOPSW2Sta_flg/1 -> STOPBELL/5(VINP_ZFRBCMSTOPSW2Sta_flg)
  DoorControl/1(VBCM_FDCBCMOutDoorOpenSWSta_enum) -> VBCM_FDCBCMOSDrOpenSWSta_enum/1
  RoomLamp/2(VBCM_FDCBCMRoomLpAmbSetSta_flg) -> VBCM_FDCBCMRoomLpAmbSetSta_flg/1
  VINP_ZRRBCMCallingSWSta_flg/1 -> STOPBELL/6(VINP_ZFRBCMCallingSWSta_flg)
  VINP_EmExitSW_flg/1 -> [VINP_EmExitSW_flg]
  RoomLamp/1(VBCM_FDCBCMRoomLpAmbCmd_flg) -> VBCM_FDCBCMRoomLpAmbCmd_flg/1
  VINP_BCUTimeout_flg/1 -> BSDandInnerBuzzer/11(VINP_BCUTimeout_flg)
  ExteriorLight/1(LBeam) -> VBCM_FDCBCMLBeamCmd_flg/1
  DoorControl/6(VBCM_FDCBCMMDCloseSVCmd_flg) -> VBCM_FDCBCMMDCloseSVCmd_flg/1
  ExteriorLight/6(RFLamp) -> VBCM_FDCBCMRFLampCmd_flg/1
  VINP_RDSW_flg/1 -> [VINP_RDSW_flg]
  VINP_EEPFDCBCMRoomLpAmbSetSta_flg/1 -> RoomLamp/3(VINP_EEPFDCBCMRoomLpAmbSetSta_flg)
  VINP_B2VFaultCode_enum/1 -> BSDandInnerBuzzer/10(VINP_B2VFaultCode_enum)
  RoomLamp/7(VBCM_FDCBCMMRoomLpCmd_pct) -> VBCM_FDCBCMMRoomLpCmd_pct/1
  DoorControl/4(VBCM_FDCBCMFDCloseSVCmd_flg) -> VBCM_FDCBCMFDCloseSVCmd_flg/1
  Constant/1 -> Data Type Conversion/1
  [VINP_FDSW_flg] -> Logical Operator6/1
  [IG1] -> BSDandInnerBuzzer/1(IG1)
  VINP_ZRRBCMRRTurnLpCSta_A/1 -> FlasherSignal/14(VINP_ZRRBCMRRTurnLpCSta_A)
  VINP_ZFRBCMRFTurnLpCSta_A/1 -> FlasherSignal/13(VINP_ZFRBCMRFTurnLpCSta_A)
  VINP_ZRRBCMLRTurnLpCSta_A/1 -> FlasherSignal/12(VINP_ZRRBCMLRTurnLpCSta_A)
  VINP_ZFRBCMLFTurnLpCSta_A/1 -> FlasherSignal/11(VINP_ZFRBCMLFTurnLpCSta_A)
  Relational Operator/1 -> Logical Operator/2
  Relational Operator1/1 -> Logical Operator/1
  Constant2/1 -> Data Type Conversion2/1
  Data Type Conversion2/1 -> Relational Operator1/1
  Logical Operator/1 -> [IG1]
  Data Type Conversion3/1 -> VBCM_FDCBCMBrakeCmd_flg/1

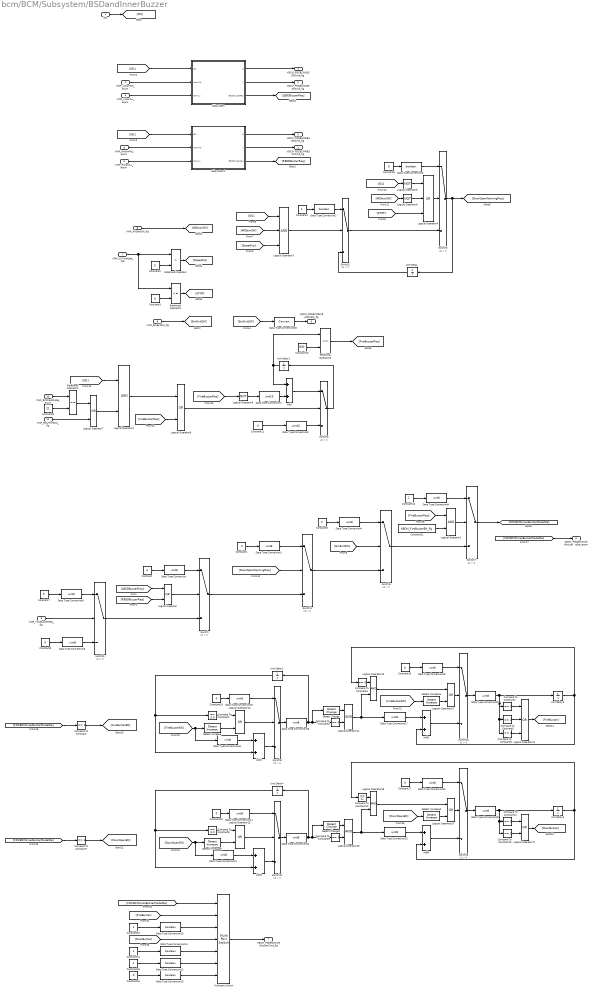
== system bcm/BCM/Subsystem/BSDandInnerBuzzer ==
  IG1 : Inport
  VINP_LWarnMd_enum : Inport  Port=2
  VINP_RWarnMd_enum : Inport  Port=3
  VINP_LWarnLv_enum : Inport  Port=4
  VINP_RWarnLv_enum : Inport  Port=5
  VINP_AllDoorSW_flg : Inport  Port=6
  VDIP_VCUVehSpd_kph : Inport  Port=7
  VINP_EmExitSW_flg : Inport  Port=8
  VINP_VCUBuzzerReq_flg : Inport  Port=9
  VINP_B2VFaultCode_enum : Inport  Port=10
  VINP_BCUTimeout_flg : Inport  Port=11
  Add{,1..4} (5 alike) : Sum
  Compare To Constant : simulink/Logic and Bit Operations/Compare To Constant  relop===  const=1  OutDataTypeStr=boolean
  Compare To Constant1 : simulink/Logic and Bit Operations/Compare To Constant  relop===  const=3.0  OutDataTypeStr=boolean
  Compare To Constant10 : simulink/Logic and Bit Operations/Compare To Constant  relop===  const=12  OutDataTypeStr=boolean
  Compare To Constant{2,4,9,11} (4 alike) : simulink/Logic and Bit Operations/Compare To Constant  relop===  const=0  OutDataTypeStr=boolean
  Compare To Constant12 : simulink/Logic and Bit Operations/Compare To Constant  relop===  const=2  OutDataTypeStr=boolean
  Compare To Constant3 : simulink/Logic and Bit Operations/Compare To Constant  relop===  const=6  OutDataTypeStr=boolean
  Compare To Constant5 : simulink/Logic and Bit Operations/Compare To Constant  relop===  const=2  OutDataTypeStr=boolean
  Compare To Constant6 : simulink/Logic and Bit Operations/Compare To Constant  relop===  const=4  OutDataTypeStr=boolean
  Compare To Constant7 : simulink/Logic and Bit Operations/Compare To Constant  relop===  const=3  OutDataTypeStr=boolean
  Compare To Constant8 : simulink/Logic and Bit Operations/Compare To Constant  relop===  const=3.0  OutDataTypeStr=boolean
  Constant : Constant  Value=4
  Constant1 : Constant  Value=3
  Constant10 : Constant  Value=800
  Constant{3,5,8,11,16..20} (9 alike) : Constant  Value=0
  Constant{4,12..15} (5 alike) : Constant
  Constant2 : Constant  Value=5
  Constant21 : Constant  Value=KBCM_FireBuzzerEN_flg
  Constant6 : Constant  Value=2
  Constant7 : Constant  Value=5
  Constant9 : Constant  Value=21
  Data Type Conversion{,1,4..6,9,14..25} (18 alike) : DataTypeConversion  OutDataTypeStr=uint8
  Data Type Conversion{2..3,10..13} (6 alike) : DataTypeConversion  OutDataTypeStr=boolean
  Data Type Conversion26 : DataTypeConversion
  Data Type Conversion7 : DataTypeConversion  OutDataTypeStr=uint16
  Data Type Conversion8 : DataTypeConversion  OutDataTypeStr=uint16
  Detect Change : simulink/Logic and Bit Operations/Detect Change  vinit=0  OutDataTypeStr=boolean
  Detect Change1 : simulink/Logic and Bit Operations/Detect Change  vinit=0  OutDataTypeStr=boolean
  Detect Increase{,1..3} (4 alike) : simulink/Logic and Bit Operations/Detect Increase  vinit=0.0  OutDataTypeStr=boolean
  Logical Operator{,7..8,10,14..15,17,19} (8 alike) : Logic  Operator=OR  AllPortsSameDT=off  OutDataTypeStr=boolean
  Logical Operator{1..2,11,13,16,18} (6 alike) : Logic  AllPortsSameDT=off  OutDataTypeStr=boolean
  Logical Operator12 : Logic  Operator=OR  Inputs=3  AllPortsSameDT=off  OutDataTypeStr=boolean
  Logical Operator3 : Logic  Inputs=3  AllPortsSameDT=off  OutDataTypeStr=boolean
  Logical Operator4 : Logic  Operator=OR  Inputs=3  AllPortsSameDT=off  OutDataTypeStr=boolean
  Logical Operator5 : Logic  Operator=NOT  AllPortsSameDT=off  OutDataTypeStr=boolean
  Logical Operator6 : Logic  Operator=NOT  AllPortsSameDT=off  OutDataTypeStr=boolean
  Logical Operator9 : Logic  Operator=NOT  AllPortsSameDT=off  OutDataTypeStr=boolean
  Multiport Switch : MultiPortSwitch  Inputs=5  DataPortForDefault=Additional data port  DiagnosticForDefault=None
  Relational Operator : RelationalOperator  Operator=>  OutDataTypeStr=boolean  RndMeth=Simplest
  Relational Operator1 : RelationalOperator  Operator=<=  OutDataTypeStr=boolean  RndMeth=Simplest
  Relational Operator2 : RelationalOperator  Operator===  OutDataTypeStr=boolean  RndMeth=Simplest
  Relational Operator3 : RelationalOperator  OutDataTypeStr=boolean  RndMeth=Simplest
  Subsystem : Subsystem
  Subsystem1 : Subsystem
  Switch{,1..11} (12 alike) : Switch  Criteria=u2 > Threshold
  Unit Delay{,1..5} (6 alike) : UnitDelay  SampleTime=-1  HasFrameUpgradeWarning=on
  VBCM_FDCBCMLBSDRCmd_flg : Outport
  VBCM_FDCBCMLBSDYCmd_flg : Outport  Port=2
  VBCM_FDCBCMRBSDRCmd_flg : Outport  Port=3
  VBCM_FDCBCMRBSDYCmd_flg : Outport  Port=4
  VBCM_FDCBCMEmExitSWSta_flg : Outport  Port=5
  VBCM_FDCBCMInnerBuzzerModeSta_enum : Outport  Port=6
  VBCM_FDCBCMInnerBuzzerCmd_flg : Outport  Port=7
  wires:
  IG1/1 -> [IG1]
  VINP_LWarnMd_enum/1 -> Subsystem/2(WarnMd)
  VINP_LWarnLv_enum/1 -> Subsystem/3(WarnLv)
  VINP_RWarnMd_enum/1 -> Subsystem1/2(WarnMd)
  VINP_RWarnLv_enum/1 -> Subsystem1/3(WarnLv)
  Subsystem/1(R) -> VBCM_FDCBCMLBSDRCmd_flg/1
  Subsystem/2(Y) -> VBCM_FDCBCMLBSDYCmd_flg/1
  Subsystem1/1(R) -> VBCM_FDCBCMRBSDRCmd_flg/1
  Subsystem1/2(Y) -> VBCM_FDCBCMRBSDYCmd_flg/1
  [IG1] -> Subsystem/1(IG1)
  [IG1] -> Subsystem1/1(IG1)
  Subsystem/3(BSDBuzzerReq) -> [LBSDBuzzerReq]
  Subsystem1/3(BSDBuzzerReq) -> [RBSDBuzzerReq]
  [LBSDBuzzerReq] -> Logical Operator/1
  [RBSDBuzzerReq] -> Logical Operator/2
  Logical Operator/1 -> Switch/2
  Data Type Conversion/1 -> Switch/1
  Constant/1 -> Data Type Conversion/1
  Constant1/1 -> Data Type Conversion1/1
  Data Type Conversion1/1 -> Switch1/1
  VINP_AllDoorSW_flg/1 -> [AllDoorSW]
  VDIP_VCUVehSpd_kph/1 -> Relational Operator1/1, Relational Operator/1
  Constant2/1 -> Relational Operator/2
  Constant3/1 -> Relational Operator1/2
  [IG1] -> Logical Operator3/1
  [AllDoorSW] -> Logical Operator3/2
  Relational Operator/1 -> [SpeedUp]
  [SpeedUp] -> Logical Operator3/3
  Logical Operator3/1 -> Switch2/2
  Data Type Conversion2/1 -> Switch2/1
  Constant4/1 -> Data Type Conversion2/1
  Switch2/1 -> Switch3/3
  Logical Operator4/1 -> Switch3/2
  [STOP] -> Logical Operator4/3
  [IG1] -> Logical Operator5/1
  Logical Operator5/1 -> Logical Operator4/1
  Logical Operator6/1 -> Logical Operator4/2
  [AllDoorSW] -> Logical Operator6/1
  Constant5/1 -> Data Type Conversion3/1
  Data Type Conversion3/1 -> Switch3/1
  Unit Delay/1 -> Switch2/3
  Switch3/1 -> [DoorOpenWarningReq], Unit Delay/1
  [DoorOpenWarningReq] -> Switch1/2
  Switch/1 -> Switch1/3
  Switch1/1 -> Switch4/3
  Relational Operator1/1 -> [STOP]
  VINP_EmExitSW_flg/1 -> [EmExitSW]
  [EmExitSW] -> Data Type Conversion26/1
  [EmExitSW] -> Switch4/2
  Data Type Conversion4/1 -> Switch4/1
  Constant6/1 -> Data Type Conversion4/1
  Switch5/1 -> Switch/3
  VINP_VCUBuzzerReq_flg/1 -> Switch5/2
  Constant7/1 -> Data Type Conversion5/1
  Data Type Conversion5/1 -> Switch5/1
  Data Type Conversion6/1 -> Switch5/3
  Constant8/1 -> Data Type Conversion6/1
  [IG1] -> Logical Operator1/1
  VINP_B2VFaultCode_enum/1 -> Relational Operator2/1
  Constant9/1 -> Relational Operator2/2
  Relational Operator2/1 -> Logical Operator7/1
  VINP_BCUTimeout_flg/1 -> Logical Operator7/2
  Logical Operator7/1 -> Logical Operator1/2
  Logical Operator1/1 -> Logical Operator8/1
  Logical Operator8/1 -> Switch6/2
  Add/1 -> Switch6/1
  Unit Delay1/1 -> Relational Operator3/1, Add/1
  Constant10/1 -> Relational Operator3/2
  Data Type Conversion7/1 -> Add/2
  Switch6/1 -> Unit Delay1/1
  Data Type Conversion8/1 -> Switch6/3
  Constant11/1 -> Data Type Conversion8/1
  Relational Operator3/1 -> [FireBuzzerReq]
  [FireBuzzerReq] -> Logical Operator8/2
  Logical Operator9/1 -> Data Type Conversion7/1
  [FireBuzzerReq] -> Logical Operator9/1
  Switch4/1 -> Switch7/3
  [FireBuzzerReq] -> Logical Operator2/1
  Constant12/1 -> Data Type Conversion9/1
  Data Type Conversion9/1 -> Switch7/1
  Switch7/1 -> [FDCBCMInnerBuzzerModeSta]
  [FDCBCMInnerBuzzerModeSta] -> VBCM_FDCBCMInnerBuzzerModeSta_enum/1
  [FDCBCMInnerBuzzerModeSta] -> Multiport Switch/1
  Constant13/1 -> Data Type Conversion10/1
  Data Type Conversion10/1 -> Multiport Switch/3
  Data Type Conversion11/1 -> Multiport Switch/5
  Constant14/1 -> Data Type Conversion11/1
  Data Type Conversion12/1 -> Multiport Switch/6
  Constant15/1 -> Data Type Conversion12/1
  Data Type Conversion13/1 -> Multiport Switch/7
  Constant16/1 -> Data Type Conversion13/1
  [FDCBCMInnerBuzzerModeSta] -> Compare To Constant/1
  Compare To Constant/1 -> [FireBuzzerEN]
  [FireBuzzerEN] -> Data Type Conversion16/1, Detect Increase/1
  Constant19/1 -> Data Type Conversion15/1
  Data Type Conversion15/1 -> Switch9/1
  Logical Operator10/1 -> Switch9/2
  Detect Increase/1 -> Logical Operator10/2
  Compare To Constant1/1 -> Logical Operator10/1
  Unit Delay2/1 -> Add1/2, Compare To Constant1/1
  Switch9/1 -> Data Type Conversion19/1
  Add1/1 -> Switch9/3
  Data Type Conversion16/1 -> Add1/1
  [FireBuzzerEN] -> Detect Increase1/1
  Detect Change/1 -> Logical Operator11/1
  Compare To Constant2/1 -> Logical Operator11/2
  Add2/1 -> Switch10/3
  Logical Operator11/1 -> Logical Operator13/2, Data Type Conversion17/1
  Data Type Conversion17/1 -> Add2/1
  Unit Delay3/1 -> Compare To Constant3/1, Add2/2
  Switch10/1 -> Data Type Conversion20/1
  Data Type Conversion18/1 -> Switch10/1
  Constant18/1 -> Data Type Conversion18/1
  Data Type Conversion19/1 -> Detect Change/1, Compare To Constant2/1, Unit Delay2/1
  Data Type Conversion20/1 -> Compare To Constant6/1, Compare To Constant5/1, Compare To Constant4/1, Unit Delay3/1
  Compare To Constant3/1 -> Logical Operator13/1
  Logical Operator14/1 -> Switch10/2
  Detect Increase1/1 -> Logical Operator14/2
  Logical Operator13/1 -> Logical Operator14/1
  Compare To Constant5/1 -> Logical Operator12/2
  Compare To Constant4/1 -> Logical Operator12/1
  Compare To Constant6/1 -> Logical Operator12/3
  Logical Operator12/1 -> [FireBuzzer]
  [FireBuzzer] -> Multiport Switch/2
  Logical Operator17/1 -> [DoorBuzzer]
  Compare To Constant11/1 -> Logical Operator17/1
  Compare To Constant12/1 -> Logical Operator17/2
  Logical Operator18/1 -> Logical Operator19/1
  Detect Increase3/1 -> Logical Operator19/2
  Logical Operator19/1 -> Switch8/2
  Compare To Constant10/1 -> Logical Operator18/1
  Data Type Conversion25/1 -> Unit Delay5/1, Compare To Constant11/1, Compare To Constant12/1
  Data Type Conversion24/1 -> Unit Delay4/1, Compare To Constant9/1, Detect Change1/1
  Constant17/1 -> Data Type Conversion23/1
  Data Type Conversion23/1 -> Switch8/1
  Switch8/1 -> Data Type Conversion25/1
  Unit Delay5/1 -> Add4/2, Compare To Constant10/1
  Data Type Conversion22/1 -> Add4/1
  Logical Operator16/1 -> Data Type Conversion22/1, Logical Operator18/2
  Add4/1 -> Switch8/3
  Compare To Constant9/1 -> Logical Operator16/2
  Detect Change1/1 -> Logical Operator16/1
  [DoorOpenEN] -> Detect Increase3/1
  Data Type Conversion21/1 -> Add3/1
  Add3/1 -> Switch11/3
  Switch11/1 -> Data Type Conversion24/1
  Unit Delay4/1 -> Compare To Constant8/1, Add3/2
  Compare To Constant8/1 -> Logical Operator15/1
  Detect Increase2/1 -> Logical Operator15/2
  Logical Operator15/1 -> Switch11/2
  Data Type Conversion14/1 -> Switch11/1
  Constant20/1 -> Data Type Conversion14/1
  [DoorOpenEN] -> Detect Increase2/1, Data Type Conversion21/1
  Compare To Constant7/1 -> [DoorOpenEN]
  [FDCBCMInnerBuzzerModeSta] -> Compare To Constant7/1
  [DoorBuzzer] -> Multiport Switch/4
  Multiport Switch/1 -> VBCM_FDCBCMInnerBuzzerCmd_flg/1
  Logical Operator2/1 -> Switch7/2
  Constant21/1 -> Logical Operator2/2
  Data Type Conversion26/1 -> VBCM_FDCBCMEmExitSWSta_flg/1

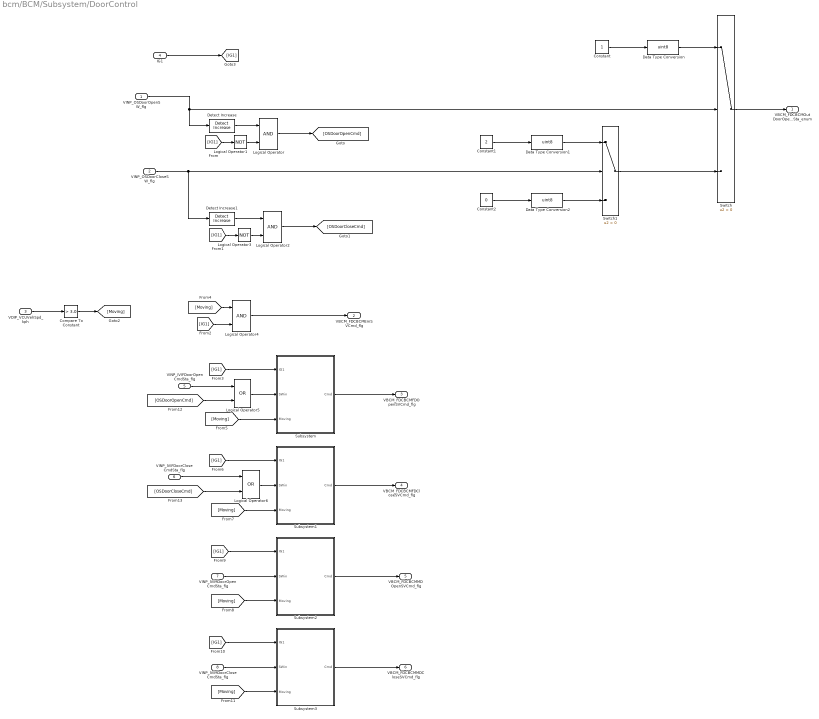
== system bcm/BCM/Subsystem/DoorControl ==
  VINP_OSDoorOpenSW_flg : Inport
  VINP_OSDoorCloseSW_flg : Inport  Port=2
  VDIP_VCUVehSpd_kph : Inport  Port=3
  IG1 : Inport  Port=4
  VINP_IVIFDoorOpenCmdSta_flg : Inport  Port=5
  VINP_IVIFDoorCloseCmdSta_flg : Inport  Port=6
  VINP_IVIMDoorOpenCmdSta_flg : Inport  Port=7
  VINP_IVIMDoorCloseCmdSta_flg : Inport  Port=8
  Compare To Constant : simulink/Logic and Bit Operations/Compare To Constant  relop=>  const=3.0  OutDataTypeStr=boolean
  Constant : Constant
  Constant1 : Constant  Value=2
  Constant2 : Constant  Value=0
  Data Type Conversion : DataTypeConversion  OutDataTypeStr=uint8
  Data Type Conversion1 : DataTypeConversion  OutDataTypeStr=uint8
  Data Type Conversion2 : DataTypeConversion  OutDataTypeStr=uint8
  Detect Increase : simulink/Logic and Bit Operations/Detect Increase  vinit=0.0  OutDataTypeStr=boolean
  Detect Increase1 : simulink/Logic and Bit Operations/Detect Increase  vinit=0.0  OutDataTypeStr=boolean
  Logical Operator : Logic  AllPortsSameDT=off  OutDataTypeStr=boolean
  Logical Operator1 : Logic  Operator=NOT  AllPortsSameDT=off  OutDataTypeStr=boolean
  Logical Operator2 : Logic  AllPortsSameDT=off  OutDataTypeStr=boolean
  Logical Operator3 : Logic  Operator=NOT  AllPortsSameDT=off  OutDataTypeStr=boolean
  Logical Operator4 : Logic  AllPortsSameDT=off  OutDataTypeStr=boolean
  Logical Operator5 : Logic  Operator=OR  AllPortsSameDT=off  OutDataTypeStr=boolean
  Logical Operator6 : Logic  Operator=OR  AllPortsSameDT=off  OutDataTypeStr=boolean
  Subsystem : Subsystem
  Subsystem1 : Subsystem
  Subsystem2 : Subsystem
  Subsystem3 : Subsystem
  Switch : Switch  Criteria=u2 > Threshold
  Switch1 : Switch  Criteria=u2 > Threshold
  VBCM_FDCBCMOutDoorOpenSWSta_enum : Outport
  VBCM_FDCBCMEmSVCmd_flg : Outport  Port=2
  VBCM_FDCBCMFDOpenSVCmd_flg : Outport  Port=3
  VBCM_FDCBCMFDCloseSVCmd_flg : Outport  Port=4
  VBCM_FDCBCMMDOpenSVCmd_flg : Outport  Port=5
  VBCM_FDCBCMMDCloseSVCmd_flg : Outport  Port=6
  wires:
  VINP_OSDoorOpenSW_flg/1 -> Detect Increase/1, Switch/2
  VINP_OSDoorCloseSW_flg/1 -> Detect Increase1/1, Switch1/2
  Logical Operator/1 -> [OSDoorOpenCmd]
  VDIP_VCUVehSpd_kph/1 -> Compare To Constant/1
  IG1/1 -> [IG1]
  Detect Increase/1 -> Logical Operator/1
  Logical Operator1/1 -> Logical Operator/2
  [IG1] -> Logical Operator1/1
  Detect Increase1/1 -> Logical Operator2/1
  [IG1] -> Logical Operator3/1
  Logical Operator3/1 -> Logical Operator2/2
  Logical Operator2/1 -> [OSDoorCloseCmd]
  Compare To Constant/1 -> [Moving]
  [IG1] -> Logical Operator4/2
  Logical Operator4/1 -> VBCM_FDCBCMEmSVCmd_flg/1
  [Moving] -> Logical Operator4/1
  [Moving] -> Subsystem/3(Moving)
  [IG1] -> Subsystem/1(IG1)
  VINP_IVIFDoorOpenCmdSta_flg/1 -> Logical Operator5/1
  Subsystem/1(Cmd) -> VBCM_FDCBCMFDOpenSVCmd_flg/1
  Subsystem1/1(Cmd) -> VBCM_FDCBCMFDCloseSVCmd_flg/1
  [IG1] -> Subsystem1/1(IG1)
  [Moving] -> Subsystem1/3(Moving)
  Subsystem2/1(Cmd) -> VBCM_FDCBCMMDOpenSVCmd_flg/1
  VINP_IVIMDoorOpenCmdSta_flg/1 -> Subsystem2/2(SWin)
  [Moving] -> Subsystem2/3(Moving)
  [IG1] -> Subsystem2/1(IG1)
  Subsystem3/1(Cmd) -> VBCM_FDCBCMMDCloseSVCmd_flg/1
  VINP_IVIMDoorCloseCmdSta_flg/1 -> Subsystem3/2(SWin)
  [IG1] -> Subsystem3/1(IG1)
  [Moving] -> Subsystem3/3(Moving)
  Logical Operator5/1 -> Subsystem/2(SWin)
  [OSDoorOpenCmd] -> Logical Operator5/2
  Logical Operator6/1 -> Subsystem1/2(SWin)
  VINP_IVIFDoorCloseCmdSta_flg/1 -> Logical Operator6/1
  [OSDoorCloseCmd] -> Logical Operator6/2
  Switch/1 -> VBCM_FDCBCMOutDoorOpenSWSta_enum/1
  Data Type Conversion/1 -> Switch/1
  Constant/1 -> Data Type Conversion/1
  Switch1/1 -> Switch/3
  Constant1/1 -> Data Type Conversion1/1
  Data Type Conversion1/1 -> Switch1/1
  Data Type Conversion2/1 -> Switch1/3
  Constant2/1 -> Data Type Conversion2/1

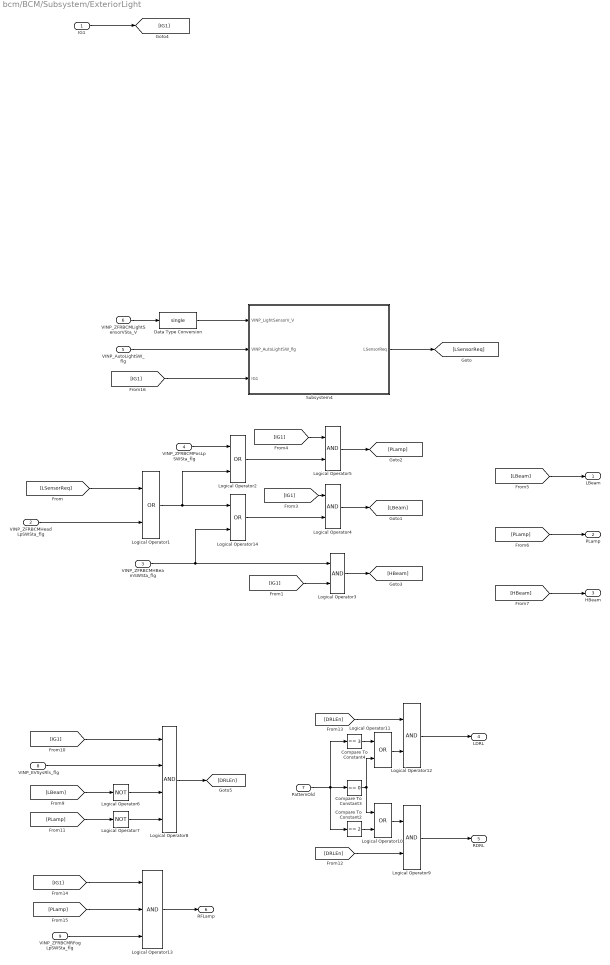
== system bcm/BCM/Subsystem/ExteriorLight ==
  IG1 : Inport
  VINP_ZFRBCMHeadLpSWSta_flg : Inport  Port=2
  VINP_ZFRBCMHBeamSWSta_flg : Inport  Port=3
  VINP_ZFRBCMPosLpSWSta_flg : Inport  Port=4
  VINP_AutoLightSW_flg : Inport  Port=5
  VINP_ZFRBCMLightSensorVSta_V : Inport  Port=6
  PatternOld : Inport  Port=7
  VINP_EVSysRls_flg : Inport  Port=8
  VINP_ZFRBCMRFogLpSWSta_flg : Inport  Port=9
  Compare To Constant2 : simulink/Logic and Bit Operations/Compare To Constant  relop===  const=2  OutDataTypeStr=boolean
  Compare To Constant3 : simulink/Logic and Bit Operations/Compare To Constant  relop===  const=0  OutDataTypeStr=boolean
  Compare To Constant4 : simulink/Logic and Bit Operations/Compare To Constant  relop===  const=3  OutDataTypeStr=boolean
  Data Type Conversion : DataTypeConversion  OutDataTypeStr=single
  Logical Operator{1..2,10..11,14} (5 alike) : Logic  Operator=OR  AllPortsSameDT=off  OutDataTypeStr=boolean
  Logical Operator{3..5,9,12} (5 alike) : Logic  AllPortsSameDT=off  OutDataTypeStr=boolean
  Logical Operator13 : Logic  Inputs=3  AllPortsSameDT=off  OutDataTypeStr=boolean
  Logical Operator6 : Logic  Operator=NOT  AllPortsSameDT=off  OutDataTypeStr=boolean
  Logical Operator7 : Logic  Operator=NOT  AllPortsSameDT=off  OutDataTypeStr=boolean
  Logical Operator8 : Logic  Inputs=4  AllPortsSameDT=off  OutDataTypeStr=boolean
  Subsystem4 : Subsystem
  LBeam : Outport
  PLamp : Outport  Port=2
  HBeam : Outport  Port=3
  LDRL : Outport  Port=4
  RDRL : Outport  Port=5
  RFLamp : Outport  Port=6
  wires:
  Logical Operator4/1 -> [LBeam]
  VINP_AutoLightSW_flg/1 -> Subsystem4/2(VINP_AutoLightSW_flg)
  Logical Operator5/1 -> [PLamp]
  [IG1] -> Logical Operator4/1
  Logical Operator1/1 -> Logical Operator14/1, Logical Operator2/2
  VINP_ZFRBCMHeadLpSWSta_flg/1 -> Logical Operator1/2
  Logical Operator2/1 -> Logical Operator5/2
  Logical Operator3/1 -> [HBeam]
  [IG1] -> Logical Operator5/1
  [LSensorReq] -> Logical Operator1/1
  IG1/1 -> [IG1]
  [LBeam] -> LBeam/1
  [PLamp] -> PLamp/1
  [HBeam] -> HBeam/1
  VINP_ZFRBCMLightSensorVSta_V/1 -> Data Type Conversion/1
  [LBeam] -> Logical Operator6/1
  [PLamp] -> Logical Operator7/1
  [IG1] -> Logical Operator8/1
  VINP_EVSysRls_flg/1 -> Logical Operator8/2
  Logical Operator7/1 -> Logical Operator8/4
  Logical Operator6/1 -> Logical Operator8/3
  Logical Operator8/1 -> [DRLEn]
  [DRLEn] -> Logical Operator9/2
  PatternOld/1 -> Compare To Constant4/1, Compare To Constant3/1, Compare To Constant2/1
  Compare To Constant2/1 -> Logical Operator10/2
  Logical Operator10/1 -> Logical Operator9/1
  Compare To Constant3/1 -> Logical Operator11/2, Logical Operator10/1
  Compare To Constant4/1 -> Logical Operator11/1
  Logical Operator11/1 -> Logical Operator12/2
  [DRLEn] -> Logical Operator12/1
  Logical Operator12/1 -> LDRL/1
  Logical Operator9/1 -> RDRL/1
  [PLamp] -> Logical Operator13/2
  [IG1] -> Logical Operator13/1
  VINP_ZFRBCMRFogLpSWSta_flg/1 -> Logical Operator13/3
  Logical Operator13/1 -> RFLamp/1
  Data Type Conversion/1 -> Subsystem4/1(VINP_LightSensorV_V)
  [IG1] -> Subsystem4/3(IG1)
  Subsystem4/1(LSensorReq) -> [LSensorReq]
  VINP_ZFRBCMPosLpSWSta_flg/1 -> Logical Operator2/1
  VINP_ZFRBCMHBeamSWSta_flg/1 -> Logical Operator3/1, Logical Operator14/2
  [IG1] -> Logical Operator3/2
  Logical Operator14/1 -> Logical Operator4/2
